simulink model "simulink_non"  (R2015b)
settings: Solver=FixedStepAuto  StartTime=0.0  StopTime=30  FixedStep=0.1  RelTol=1e-3
settings Model: Creator=guilh_000  LastModifiedBy=guilh_000

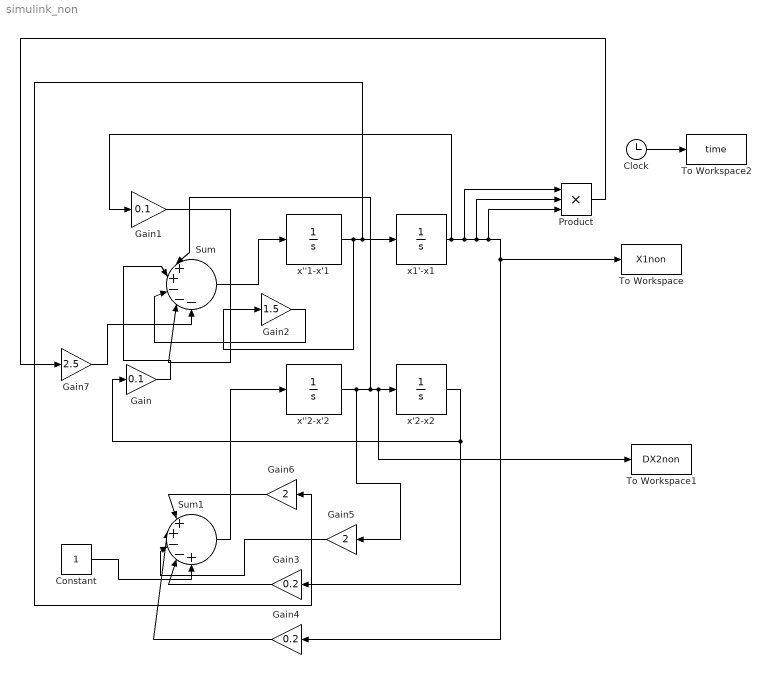
== system simulink_non ==
  Clock : Clock
  Constant : Constant
  Gain : Gain  Gain=0.1
  Gain1 : Gain  Gain=0.1
  Gain2 : Gain  Gain=1.5
  Gain3 : Gain  Gain=0.2
  Gain4 : Gain  Gain=0.2
  Gain5 : Gain  Gain=2
  Gain6 : Gain  Gain=2
  Gain7 : Gain  Gain=2.5
  Product : Product  Inputs=3
  Sum : Sum  Inputs=|++---
  Sum1 : Sum  Inputs=|++--+
  To Workspace : ToWorkspace  VariableName=X1non  SampleTime=-1
  To Workspace1 : ToWorkspace  VariableName=DX2non  SampleTime=-1
  To Workspace2 : ToWorkspace  VariableName=time  SampleTime=-1
  x''1-x'1 : Integrator
  x''2-x'2 : Integrator
  x'2-x2 : Integrator
  x1'-x1 : Integrator
  wires:
  Sum/1 -> x''1-x'1/1
  x''1-x'1/1 -> Gain2/1, Gain6/1, x1'-x1/1
  Sum1/1 -> x''2-x'2/1
  x''2-x'2/1 -> Gain5/1, Sum/1, To Workspace1/1, x'2-x2/1
  x'2-x2/1 -> Gain3/1, Gain/1
  Gain/1 -> Sum/2
  Gain1/1 -> Sum/4
  Gain2/1 -> Sum/3
  Gain3/1 -> Sum1/4
  Gain4/1 -> Sum1/2
  x1'-x1/1 -> Gain1/1, Product/1, Product/2, Product/3, To Workspace/1, Gain4/1
  Gain5/1 -> Sum1/3
  Gain6/1 -> Sum1/1
  Clock/1 -> To Workspace2/1
  Product/1 -> Gain7/1
  Gain7/1 -> Sum/5
  Constant/1 -> Sum1/5
